simulink model "full_model_openLoop"  (R2022a)
settings: Solver=ode23s  StartTime=0.0  StopTime=t_end  RelTol=1e-9  AbsTol=1e-9
undefined symbols (not defined in the file): omega_0, paramStruct, theta_0
settings Model: PauseTimes=0  Creator=Philipp  LastModifiedBy=Philipp
settings DebuggingCC: UnconnectedInputMsg=warning  UnconnectedOutputMsg=warning  UnconnectedLineMsg=warning  UnderSpecifiedDimensionMsg=warning
settings ModelReferenceCC: ModelReferenceMinAlgLoopOccurrences=on
settings RTWCC: DLArmComputeVersion=19.05

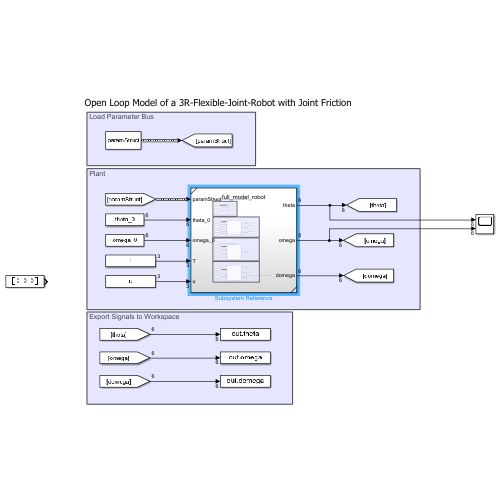
[thumbnail: Simulink's stored preview of the top-level diagram]
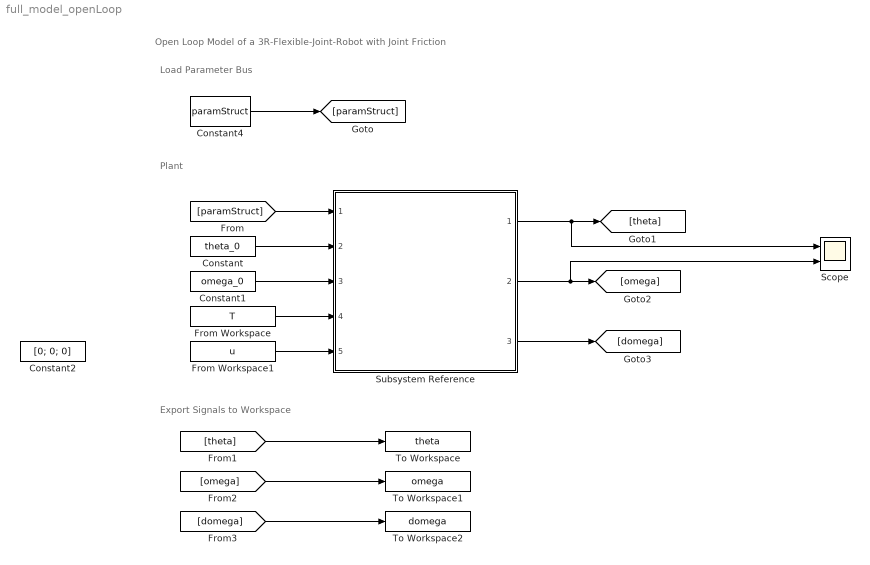
== system full_model_openLoop ==
  note: Export Signals to Workspace
  note: Load Parameter Bus
  note: Plant
  note: Open Loop Model of a 3R-Flexible-Joint-Robot with Joint Friction
  Constant : Constant  Value=theta_0
  Constant1 : Constant  Value=omega_0
  Constant2 : Constant  Value=[0; 0; 0]
  Constant4 : Constant  InitFcn=|  Value=paramStruct  OutDataTypeStr=Bus: main_bus
      | % Import MATLAB evalin command
      | eml.extrinsic('evalin');
      | 
      | 
      | % Get contents of the structure a and output it
      | y = evalin('base', 'paramStruct');
  From Workspace : FromWorkspace  VariableName=T
  From Workspace1 : FromWorkspace  VariableName=u
  Scope : Scope  NumInputPorts=2
  Subsystem Reference : Subsystem  ReferencedSubsystem=full_model_robot
  To Workspace : ToWorkspace  VariableName=theta  SampleTime=-1
  To Workspace1 : ToWorkspace  VariableName=omega  SampleTime=-1
  To Workspace2 : ToWorkspace  VariableName=domega  SampleTime=-1
  wires:
  Constant/1 -> Subsystem Reference/2
  Constant1/1 -> Subsystem Reference/3
  [paramStruct] -> Subsystem Reference/1
  From Workspace/1 -> Subsystem Reference/4
  Subsystem Reference/1 -> Scope/1, [theta]
  Subsystem Reference/2 -> Scope/2, [omega]
  Subsystem Reference/3 -> [domega]
  [theta] -> To Workspace/1
  [domega] -> To Workspace2/1
  [omega] -> To Workspace1/1
  Constant4/1 -> [paramStruct]
  From Workspace1/1 -> Subsystem Reference/5
